simulink model "pd_plus_testings"  (R2022b)
settings: Solver=VariableStepAuto  StartTime=0.0  StopTime=10.0  RelTol=1e-3
InitFcn:
  | parameters_7dof;
undefined symbols (not defined in the file): param_robot, q_0
settings Model: Creator=emu  LastModifiedBy=emu

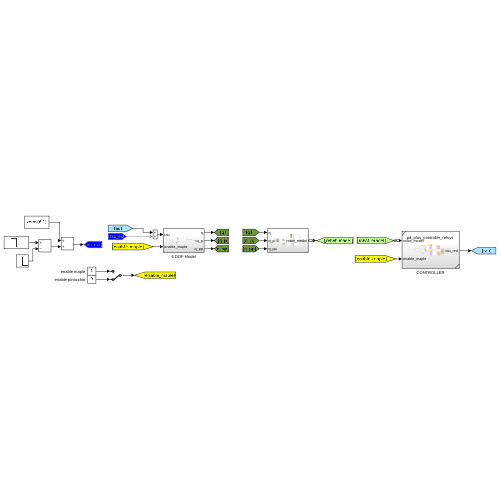
[thumbnail: Simulink's stored preview of the top-level diagram]
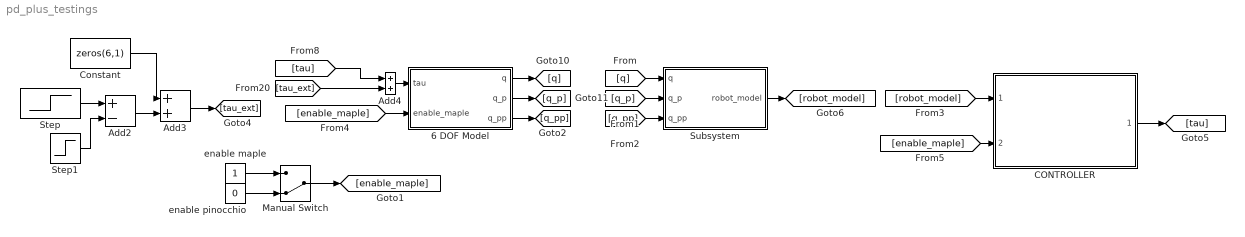
== system pd_plus_testings ==
  6 DOF Model : Subsystem
  Add2 : Sum  Inputs=+-
  Add3 : Sum
  Add4 : Sum
  CONTROLLER : Subsystem  ReferencedSubsystem=pd_plus_controller_refsys
  Constant : Constant  Value=zeros(6,1)
  Manual Switch : ManualSwitch  CurrentSetting=0
  Step : Step  Time=2  Before=1  After=0  SampleTime=0
  Step1 : Step  Before=1  After=0  SampleTime=0
  Subsystem : Subsystem
  enable maple : Constant
  enable pinocchio : Constant  Value=0
  wires:
  [q] -> Subsystem/1(q)
  [q_pp] -> Subsystem/3(q_pp)
  [q_p] -> Subsystem/2(q_p)
  [robot_model] -> CONTROLLER/1
  Step/1 -> Add2/1
  Step1/1 -> Add2/2
  Add2/1 -> Add3/2
  Constant/1 -> Add3/1
  6 DOF Model/1(q) -> [q]
  6 DOF Model/2(q_p) -> [q_p]
  6 DOF Model/3(q_pp) -> [q_pp]
  [tau] -> Add4/1
  Add4/1 -> 6 DOF Model/1(tau)
  [tau_ext] -> Add4/2
  Subsystem/1(robot_model) -> [robot_model]
  CONTROLLER/1 -> [tau]
  Add3/1 -> [tau_ext]
  enable maple/1 -> Manual Switch/1
  enable pinocchio/1 -> Manual Switch/2
  Manual Switch/1 -> [enable_maple]
  [enable_maple] -> 6 DOF Model/2(enable_maple)
  [enable_maple] -> CONTROLLER/2

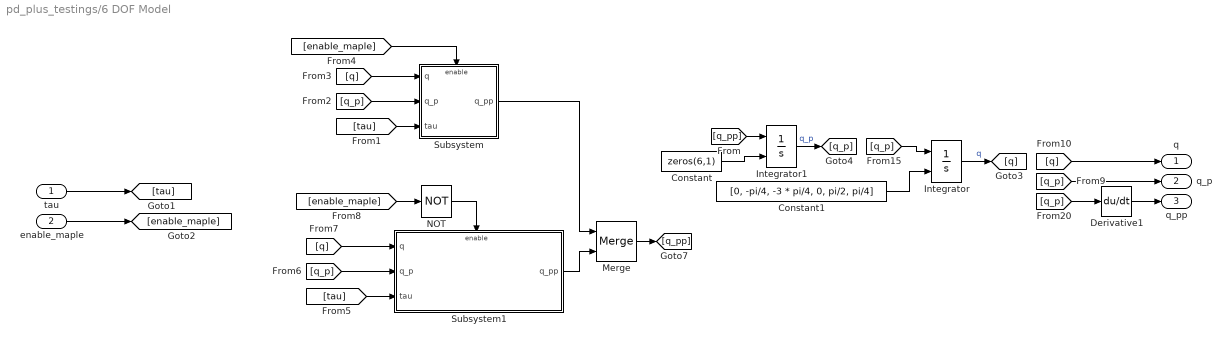
== system pd_plus_testings/6 DOF Model ==
  tau : Inport
  enable_maple : Inport  Port=2
  Constant : Constant  Value=zeros(6,1)
  Constant1 : Constant  Value=[0, -pi/4, -3 * pi/4, 0, pi/2, pi/4]
  Derivative1 : Derivative
  Integrator : Integrator  InitialConditionSource=external  InitialCondition=q_0  UpperSaturationLimit=param_robot.q_limit_upper  LowerSaturationLimit=param_robot.q_limit_lower
  Integrator1 : Integrator  InitialConditionSource=external  InitialCondition=param_robot.q_0_p_ref  UpperSaturationLimit=param_robot.q_p_limit_upper  LowerSaturationLimit=param_robot.q_p_limit_lower
  Merge : Merge
  NOT : Logic  Operator=NOT  IconShape=distinctive  AllPortsSameDT=off  OutDataTypeStr=boolean
  Subsystem : Subsystem
  Subsystem1 : Subsystem
  q : Outport
  q_p : Outport  Port=2
  q_pp : Outport  Port=3
  wires:
  [q_p] -> Derivative1/1
  Derivative1/1 -> q_pp/1
  tau/1 -> [tau]
  [q_p] -> q_p/1
  [q_p] -> Integrator/1
  Integrator1/1 -> [q_p]  "q_p"
  Integrator/1 -> [q]  "q"
  [q] -> q/1
  [q_pp] -> Integrator1/1
  Constant/1 -> Integrator1/2
  Constant1/1 -> Integrator/2
  [q] -> Subsystem/1(q)
  [q_p] -> Subsystem/2(q_p)
  [tau] -> Subsystem/3(tau)
  Subsystem/1(q_pp) -> Merge/1
  [q] -> Subsystem1/1(q)
  [q_p] -> Subsystem1/2(q_p)
  [tau] -> Subsystem1/3(tau)
  Subsystem1/1(q_pp) -> Merge/2
  Merge/1 -> [q_pp]
  NOT/1 -> Subsystem1/Enable
  enable_maple/1 -> [enable_maple]
  [enable_maple] -> NOT/1
  [enable_maple] -> Subsystem/Enable

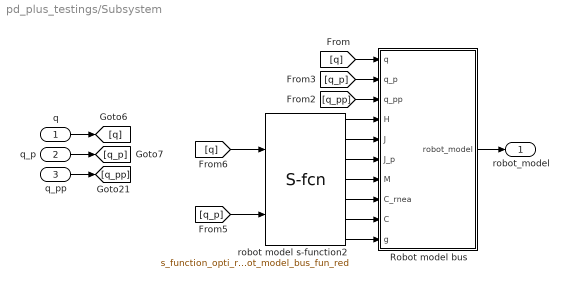
== system pd_plus_testings/Subsystem ==
  q : Inport
  q_p : Inport  Port=2
  q_pp : Inport  Port=3
  Robot model bus : MATLAB Function  TreatAsAtomicUnit=on
  robot model s-function2 : S-Function  FunctionName=s_function_opti_robot_model_bus_fun_red  SFunctionModules='robot_model_bus_fun_red'  SFunctionDeploymentMode=off  EnableBusSupport=off
  robot_model : Outport  OutDataTypeStr=Bus: robot_model_red
  wires:
  robot model s-function2/5 -> Robot model bus/8(C_rnea)
  robot model s-function2/4 -> Robot model bus/7(M)
  robot model s-function2/1 -> Robot model bus/4(H)
  [q] -> robot model s-function2/1
  robot model s-function2/2 -> Robot model bus/5(J)
  [q] -> Robot model bus/1(q)
  q_pp/1 -> [q_pp]
  [q_p] -> Robot model bus/2(q_p)
  robot model s-function2/6 -> Robot model bus/9(C)
  q_p/1 -> [q_p]
  [q_p] -> robot model s-function2/2
  robot model s-function2/7 -> Robot model bus/10(g)
  q/1 -> [q]
  [q_pp] -> Robot model bus/3(q_pp)
  robot model s-function2/3 -> Robot model bus/6(J_p)
  Robot model bus/1(robot_model) -> robot_model/1

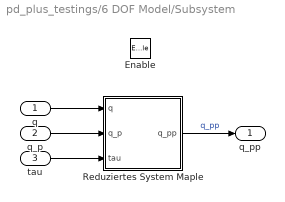
== system pd_plus_testings/6 DOF Model/Subsystem ==
  q : Inport
  q_p : Inport  Port=2
  tau : Inport  Port=3
  Enable : EnablePort
  Reduziertes System Maple : MATLAB Function
  q_pp : Outport
  wires:
  tau/1 -> Reduziertes System Maple/3(tau)
  q/1 -> Reduziertes System Maple/1(q)
  q_p/1 -> Reduziertes System Maple/2(q_p)
  Reduziertes System Maple/1(q_pp) -> q_pp/1  "q_pp"

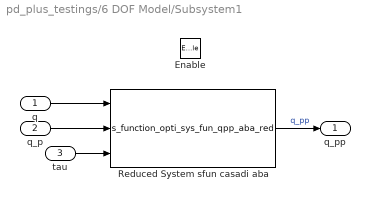
== system pd_plus_testings/6 DOF Model/Subsystem1 ==
  q : Inport
  q_p : Inport  Port=2
  tau : Inport  Port=3
  Enable : EnablePort
  Reduced System sfun casadi aba : S-Function  FunctionName=s_function_opti_sys_fun_qpp_aba_red  SFunctionModules='sys_fun_qpp_aba_red'  SFunctionDeploymentMode=off  EnableBusSupport=off
  q_pp : Outport
  wires:
  q/1 -> Reduced System sfun casadi aba/1
  tau/1 -> Reduced System sfun casadi aba/3
  q_p/1 -> Reduced System sfun casadi aba/2
  Reduced System sfun casadi aba/1 -> q_pp/1  "q_pp"

== matlab function pd_plus_testings/6 DOF Model/Subsystem/Reduziertes System Maple ==
  data: q input; q_p input; tau input; q_pp output; param_robot parameter
function q_pp =fcn(q, q_p,tau, param_robot)

n_indices = param_robot.n_indices;
qq = zeros(7,1);
qq_p = zeros(7,1);

qq(n_indices) = q;
qq_p(n_indices) = q_p;

M=inertia_matrix(qq,param_robot);                          % rigid body inertia matrix
C=coriolis_matrix(qq,qq_p,param_robot);                     % coriolis matrix
g=gravitational_forces(qq,param_robot);                    % gravitational forces

M_red = M(n_indices,n_indices);
C_red = C(n_indices,n_indices);
g_red = g(n_indices);

q_pp = M_red\(tau - C_red*q_p - g_red);

% q_pp = M\(tau-C*q_p-g - 0.5*diag(ones(7,1))*q_p(3:9)); % mit Reibung

== matlab function pd_plus_testings/Subsystem/Robot model bus ==
  settings: updateMethod=DISCRETE  sampleTime=param_global.Ta
  data: q input; q_p input; q_pp input; H input; J input; J_p input; M input; C_rnea input; C input; g input; robot_model output Bus: robot_model_red
function robot_model = fcn(q, q_p, q_pp, H, J, J_p, M, C_rnea, C, g)
% Parameters
robot_model=struct();
robot_model.q=q;                    % generalized coordinates
robot_model.q_p=q_p;                % time derivative of generalized coordinates
robot_model.q_pp=q_pp;
robot_model.H=H;
robot_model.J=J;
robot_model.J_p=J_p;
robot_model.M=M;
robot_model.C_rnea=C_rnea; % C_rnea(q, q_p) = C(q, q_p)q_p + g(q) = n(q, q_p)
robot_model.C=C;
robot_model.g=g;
end
